simulink model "Bibliotheque_PT"  (R2016b)
settings: Solver=ode45  StartTime=0.0  StopTime=10.0  RelTol=1e-3  EnableMultiTasking=on
undefined symbols (not defined in the file): D, dt, gain_accelero, gain_effort_ext, gain_encodeur_moteur_rad, gain_intensite_moteur, gain_regle_mg, gain_tension_moteur, gain_vitesse_mm_s, National_Instruments, PCIe, Vsat
libraries: sldrtlib x11, simulink x1
settings Model: Creator=user  LastModifiedBy=pt_ptsi
settings DataIOCC: LimitDataPoints=on  SaveFormat=Array  SignalLoggingSaveFormat=ModelDataLogs
settings OptimizationCC: ExpressionDepthLimit=2147483647  LifeSpan=inf
settings DebuggingCC: UnderspecifiedInitializationDetection=Classic  MergeDetectMultiDrivingBlocksExec=none  SolverPrmCheckMsg=warning  FcnCallInpInsideContextMsg=warning  StateNameClashWarn=warning  SFUnexpectedBacktrackingDiag=warning  SFNoUnconditionalDefaultTransitionDiag=warning  SFExecutionAtInitializationDiag=none
settings HardwareCC: ProdBitPerPointer=32  ProdBitPerSizeT=32  ProdBitPerPtrDiffT=32  ProdLargestAtomicFloat=None  ProdIntDivRoundTo=Undefined  ProdEndianess=Unspecified  ProdWordSize=32  ProdHWDeviceType=32-bit Generic
settings ModelReferenceCC: PropagateSignalLabelsOutOfModel=off
settings GRTTargetCC: TargetLangStandard=C89/C90 (ANSI)  GeneratePreprocessorConditionals=Disable all  CombineOutputUpdateFcns=off  GRTInterface=on
settings ConfigComp: CovMetricSettings=dw  CovHtmlReporting=on  CovSaveCumulativeToWorkspaceVar=on  CovSaveSingleToWorkspaceVar=on  CovExternalEMLEnable=off  CovSFcnEnable=off

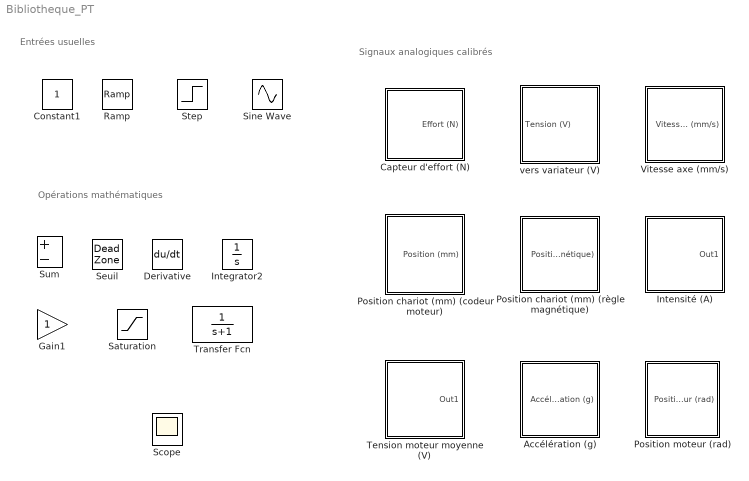
== system Bibliotheque_PT ==
  note: Signaux analogiques calibrés
  note: Opérations mathématiques
  note: Entrées usuelles
  Accélération (g) : Subsystem
      mask Display: image(imread('carte.jpg'))
  Capteur d'effort (N) : Subsystem
      mask Display: image(imread('carte.jpg'))
  Constant1 : Constant  SampleTime=dt
  Derivative : Derivative
  Gain1 : Gain
  Integrator2 : Integrator
  Intensité (A) : Subsystem
      mask Display: image(imread('carte.jpg'))
  Position chariot (mm) (codeur moteur) : Subsystem
      mask Display: image(imread('carte.jpg'))
  Position chariot (mm) (règle magnétique) : Subsystem
      mask Display: image(imread('carte.jpg'))
  Position moteur (rad) : Subsystem
      mask Display: image(imread('carte.jpg'))
  Ramp : simulink/Sources/Ramp  slope=1  start=0  X0=0
  Saturation : Saturate
  Scope : Scope
  Seuil : DeadZone  SaturateOnIntegerOverflow=on
  Sine Wave : Sin  Amplitude=5  Frequency=2*pi
  Step : Step  SampleTime=0
  Sum : Sum  Inputs=+-
  Tension moteur moyenne (V) : Subsystem
      mask Display: image(imread('carte.jpg'))
  Transfer Fcn : TransferFcn  Denominator=[1 1]
  Vitesse axe (mm/s) : Subsystem
      mask Display: image(imread('carte.jpg'))
  vers variateur (V) : Subsystem
      mask Display: image(imread('carte.jpg'))

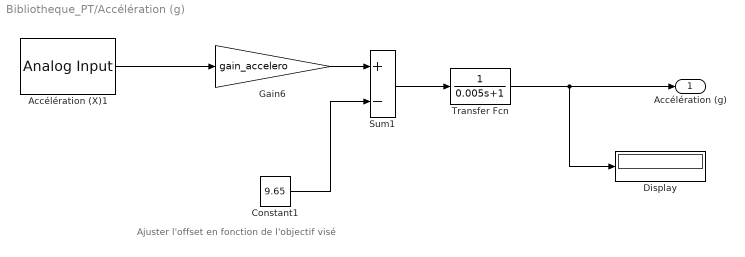
== system Bibliotheque_PT/Accélération (g) ==
  note: Ajuster l'offset en fonction de l'objectif visé
  Accélération (X)1 : sldrtlib/Analog Input  SampleTime=dt  MaxMissedTicks=10  ShowMissedTicks=off  YieldWhenWaiting=off  DrvName=National_Instruments/PCIe-6321  DrvAddress=4294967295  DrvOptions=[0 0 0 2 2 2 0]  Channels=15  RangeMode=1  VoltRange=1  DataType=1
      settings: AttributesFormatString=National Instruments\nPCIe-6321 [auto]
  Constant1 : Constant  Value=9.65  SampleTime=dt
  Display : Display
  Gain6 : Gain  Gain=gain_accelero
  Sum1 : Sum  Inputs=+-
  Transfer Fcn : TransferFcn  Denominator=[0.005 1]
  Accélération (g) : Outport
  wires:
  Accélération (X)1/1 -> Gain6/1
  Gain6/1 -> Sum1/1
  Constant1/1 -> Sum1/2
  Transfer Fcn/1 -> Display/1, Accélération (g)/1
  Sum1/1 -> Transfer Fcn/1

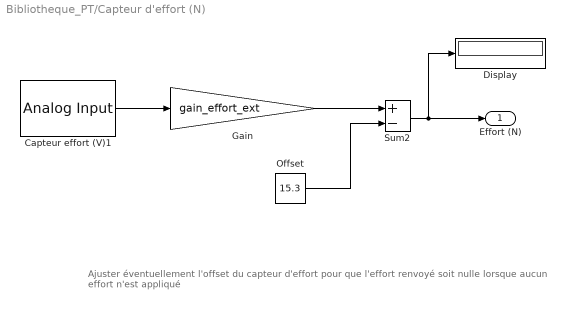
== system Bibliotheque_PT/Capteur d'effort (N) ==
  note: Ajuster éventuellement l'offset du capteur d'effort pour que
      | l'effort renvoyé soit nulle lorsque aucun effort n'est appliqué
  Capteur effort (V)1 : sldrtlib/Analog Input  SampleTime=dt  MaxMissedTicks=10  ShowMissedTicks=off  YieldWhenWaiting=off  DrvName=National_Instruments/PCIe-6321  DrvAddress=4294967295  DrvOptions=[0 0 0 2 2 2 0]  Channels=14  RangeMode=1  VoltRange=1  DataType=1
      settings: AttributesFormatString=National Instruments\nPCIe-6321 [auto]
  Display : Display
  Gain : Gain  Gain=gain_effort_ext
  Offset : Constant  Value=15.3
  Sum2 : Sum  Inputs=+-
  Effort (N) : Outport
  wires:
  Gain/1 -> Sum2/1
  Capteur effort (V)1/1 -> Gain/1
  Sum2/1 -> Display/1, Effort (N)/1
  Offset/1 -> Sum2/2

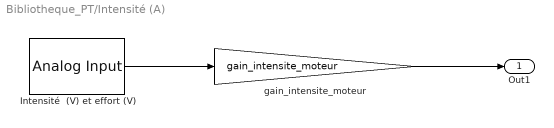
== system Bibliotheque_PT/Intensité (A) ==
  Intensité  (V) et effort (V) : sldrtlib/Analog Input  SampleTime=dt  MaxMissedTicks=10  ShowMissedTicks=off  YieldWhenWaiting=off  DrvName=National_Instruments/PCIe-6321  DrvAddress=4294967295  DrvOptions=[0 0 0 2 2 2 0]  Channels=[6]  RangeMode=1  VoltRange=1  DataType=1
      settings: AttributesFormatString=National Instruments\nPCIe-6321 [auto]
  gain_intensite_moteur : Gain  Gain=gain_intensite_moteur
  Out1 : Outport
  wires:
  gain_intensite_moteur/1 -> Out1/1
  Intensité  (V) et effort (V)/1 -> gain_intensite_moteur/1

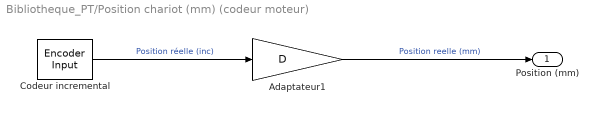
== system Bibliotheque_PT/Position chariot (mm) (codeur moteur) ==
  Adaptateur1 : Gain  Gain=D
  Codeur incremental : sldrtlib/Encoder Input  SampleTime=dt  MaxMissedTicks=10  ShowMissedTicks=off  YieldWhenWaiting=off  DrvName=National_Instruments/PCIe-6321  DrvAddress=4294967295  DrvOptions=[0 0 0 2 2 2 0]  Channels=1  QuadMode=3  IndexPulse=1  InputFilter=Inf  DataType=1
      settings: AttributesFormatString=National Instruments\nPCIe-6321 [auto]
  Position (mm) : Outport
  wires:
  Codeur incremental/1 -> Adaptateur1/1  "Position réelle (inc)"
  Adaptateur1/1 -> Position (mm)/1  "Position reelle (mm)"

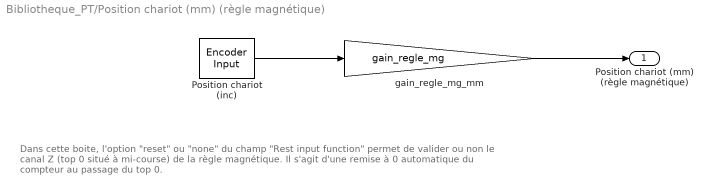
== system Bibliotheque_PT/Position chariot (mm) (règle magnétique) ==
  note: Dans cette boite, l'option "reset" ou "none" du champ "Rest input function"
      | permet de valider ou non le canal Z (top 0 situé à mi-course) de la règle magnétique.
      |
      | Il s'agit d'une remise à 0 automatique du compteur au passage du top 0.
  Position chariot (inc) : sldrtlib/Encoder Input  SampleTime=dt  MaxMissedTicks=10  ShowMissedTicks=off  YieldWhenWaiting=off  DrvName=National_Instruments/PCIe-6321  DrvAddress=4294967295  DrvOptions=[0 0 0 2 2 2 0]  Channels=2  QuadMode=3  IndexPulse=1  InputFilter=Inf  DataType=1
      settings: AttributesFormatString=National Instruments\nPCIe-6321 [auto]
  gain_regle_mg_mm : Gain  Gain=gain_regle_mg
  Position chariot (mm) (règle magnétique) : Outport
  wires:
  gain_regle_mg_mm/1 -> Position chariot (mm) (règle magnétique)/1
  Position chariot (inc)/1 -> gain_regle_mg_mm/1

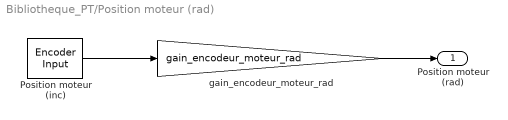
== system Bibliotheque_PT/Position moteur (rad) ==
  Position moteur (inc) : sldrtlib/Encoder Input  SampleTime=dt  MaxMissedTicks=10  ShowMissedTicks=off  YieldWhenWaiting=off  DrvName=National_Instruments/PCIe-6321  DrvAddress=4294967295  DrvOptions=[0 0 0 2 2 2 0]  Channels=1  QuadMode=3  IndexPulse=2  InputFilter=Inf  DataType=1
      settings: AttributesFormatString=National Instruments\nPCIe-6321 [auto]
  gain_encodeur_moteur_rad : Gain  Gain=gain_encodeur_moteur_rad
  Position moteur (rad) : Outport
  wires:
  gain_encodeur_moteur_rad/1 -> Position moteur (rad)/1
  Position moteur (inc)/1 -> gain_encodeur_moteur_rad/1

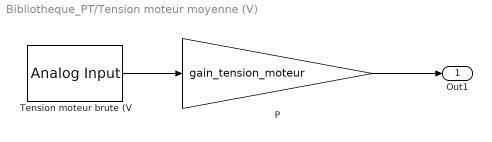
== system Bibliotheque_PT/Tension moteur moyenne (V) ==
  P : Gain  Gain=gain_tension_moteur
  "Tension moteur brute (V " : sldrtlib/Analog Input  SampleTime=dt  MaxMissedTicks=10  ShowMissedTicks=off  YieldWhenWaiting=off  DrvName=National_Instruments/PCIe-6321  DrvAddress=4294967295  DrvOptions=[0 0 0 2 2 2 0]  Channels=5  RangeMode=1  VoltRange=1  DataType=1
      settings: AttributesFormatString=National Instruments\nPCIe-6321 [auto]
  Out1 : Outport
  wires:
  "Tension moteur brute (V "/1 -> P/1
  P/1 -> Out1/1

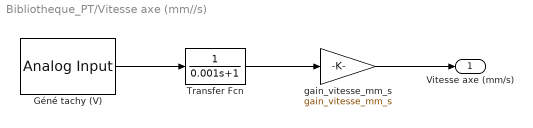
== system Bibliotheque_PT/Vitesse axe (mm//s) ==
  Géné tachy (V) : sldrtlib/Analog Input  SampleTime=dt  MaxMissedTicks=10  ShowMissedTicks=off  YieldWhenWaiting=off  DrvName=National_Instruments/PCIe-6321  DrvAddress=4294967295  DrvOptions=[0 0 0 2 2 2 0]  Channels=4  RangeMode=1  VoltRange=1  DataType=1
      settings: AttributesFormatString=National Instruments\nPCIe-6321 [auto]
  Transfer Fcn : TransferFcn  Denominator=[0.001 1]
  gain_vitesse_mm_s : Gain  Gain=gain_vitesse_mm_s
  Vitesse axe (mm/s) : Outport
  wires:
  gain_vitesse_mm_s/1 -> Vitesse axe (mm/s)/1
  Transfer Fcn/1 -> gain_vitesse_mm_s/1
  Géné tachy (V)/1 -> Transfer Fcn/1

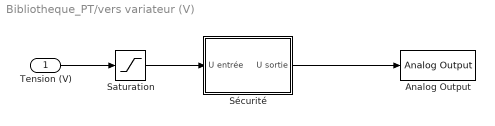
== system Bibliotheque_PT/vers variateur (V) ==
  Tension (V) : Inport
  Analog Output : sldrtlib/Analog Output  SampleTime=dt  MaxMissedTicks=10  ShowMissedTicks=off  YieldWhenWaiting=off  DrvName=National_Instruments/PCIe-6321  DrvAddress=4294967295  DrvOptions=[0 0 0 2 2 2 0]  Channels=1  RangeMode=1  VoltRange=1  InitialValue=[]  FinalValue=0
      settings: AttributesFormatString=National Instruments\nPCIe-6321 [auto]
  Saturation : Saturate  UpperLimit=10  LowerLimit=-10
  Sécurité : Subsystem
  wires:
  Sécurité/1(U sortie) -> Analog Output/1
  Saturation/1 -> Sécurité/1(U entrée)
  Tension (V)/1 -> Saturation/1

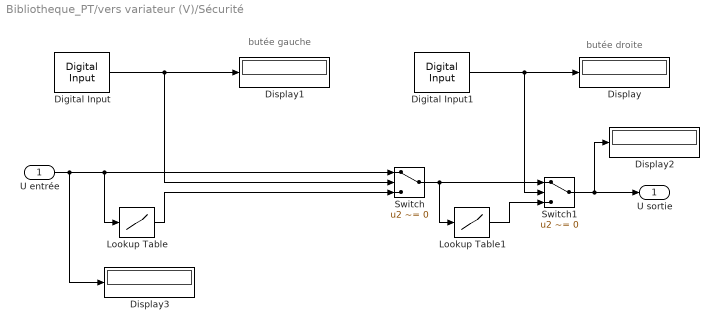
== system Bibliotheque_PT/vers variateur (V)/Sécurité ==
  note: butée gauche
  note: butée droite
  U entrée : Inport
  Digital Input : sldrtlib/Digital Input  SampleTime=dt  MaxMissedTicks=10  ShowMissedTicks=off  YieldWhenWaiting=off  DrvName=National_Instruments/PCIe-6321  DrvAddress=4294967295  DrvOptions=[0 0 0 2 2 2 0]  Channels=3  BitMode=1  DataType=9
      settings: AttributesFormatString=National Instruments\nPCIe-6321 [auto]
  Digital Input1 : sldrtlib/Digital Input  SampleTime=dt  MaxMissedTicks=10  ShowMissedTicks=off  YieldWhenWaiting=off  DrvName=National_Instruments/PCIe-6321  DrvAddress=4294967295  DrvOptions=[0 0 0 2 2 2 0]  Channels=2  BitMode=1  DataType=9
      settings: AttributesFormatString=National Instruments\nPCIe-6321 [auto]
  Display{,1..3} (4 alike) : Display
      Display settings: Decimation=3
      Display2 settings: Decimation=3
      Display3 settings: Decimation=3
  Lookup Table : Lookup  InputValues=[-Vsat 0 Vsat]  Table=[0 0 Vsat]
  Lookup Table1 : Lookup  InputValues=[-Vsat 0 Vsat]  Table=[-Vsat 0 0]
  Switch : Switch  Criteria=u2 ~= 0
  Switch1 : Switch  Criteria=u2 ~= 0
  U sortie : Outport
  wires:
  U entrée/1 -> Lookup Table/1, Switch/1, Display3/1
  Digital Input/1 -> Switch/2, Display1/1
  Lookup Table/1 -> Switch/3
  Switch/1 -> Switch1/1, Lookup Table1/1
  Digital Input1/1 -> Switch1/2, Display/1
  Lookup Table1/1 -> Switch1/3
  Switch1/1 -> U sortie/1, Display2/1
